simulink model "Lab_1b_sim"  (R2017b)
settings: Solver=VariableStepAuto  StartTime=0.0  StopTime=1.0  RelTol=1e-3
values from neighbouring files (symbols this model uses):
  alpha = 26.66667    [Lab_1.m]
  alpha_p = 32.07345    [Lab_1.m]
  beta = 133.33333    [Lab_1.m]
  K = f*(alpha_p.^2)/(4*beta)    [Lab_1.m]
  Kf = alpha_p/2    (= 16.036725)    [Lab_1.m]
settings Model: Creator=njohnson  LastModifiedBy=njohnson
settings CodeAppCC: StateflowObjectComments=on

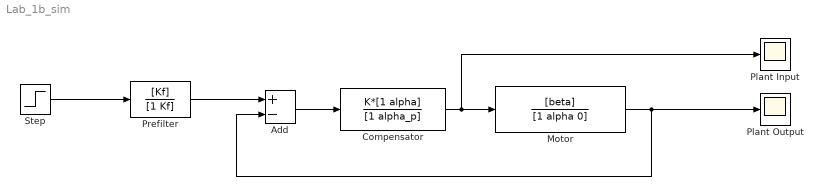
== system Lab_1b_sim ==
  Add : Sum  Inputs=+-
  "Compensator " : TransferFcn  Numerator=K*[1 alpha]  Denominator=[1 alpha_p]
  "Motor " : TransferFcn  Numerator=[beta]  Denominator=[1 alpha 0]
  Plant Input : Scope
  Plant Output : Scope
  "Prefilter " : TransferFcn  Numerator=[Kf]  Denominator=[1 Kf]
  Step : Step  Time=0  After=3  SampleTime=0
  wires:
  Add/1 -> "Compensator "/1
  "Compensator "/1 -> "Motor "/1, Plant Input/1
  "Motor "/1 -> Add/2, Plant Output/1
  Step/1 -> "Prefilter "/1
  "Prefilter "/1 -> Add/1
